simulink model "final"  (R2015a)
settings: Solver=FixedStepDiscrete  SolverMode=SingleTasking  StartTime=0.0  StopTime=3  RelTol=1e-3
PreLoadFcn:
  | Ts_Power=1e-6
  | Ts_Control=100e-6
values from neighbouring files (symbols this model uses):
  Iph_array = Iph*Npar    (= 29.801)    [sunpower305.m]
  Isat_array = Isat*Npar    (= 5.8765e-08)    [sunpower305.m]
  Rp_array = Rp*Nser/Npar    (= 198.702)    [sunpower305.m]
  Rs_array = Rs*Nser/Npar    (= 0.0075996)    [sunpower305.m]
  Ts = Ts_Power    (= 1e-06)    [sunpower305.m]
  VT_array = VT*Nser    (= 3.20466023218)    [sunpower305.m]
undefined symbols (not defined in the file or in its folder): D1, Delta, level, sigbuilder_block
libraries: powerlib x29, powerlib_extras x6, simulink x4
(part 1 of 2)
settings Model: SimulationMode=accelerator  Creator=Rupesh  LastModifiedBy=Limon
settings DataIOCC: SignalLoggingSaveFormat=ModelDataLogs
settings OptimizationCC: ExpressionDepthLimit=2147483647
settings DebuggingCC: UnderspecifiedInitializationDetection=Classic  MergeDetectMultiDrivingBlocksExec=none  SolverPrmCheckMsg=warning  FcnCallInpInsideContextMsg=EnableAllAsWarning  StateNameClashWarn=warning
settings GRTTargetCC: CombineOutputUpdateFcns=off  GRTInterface=on

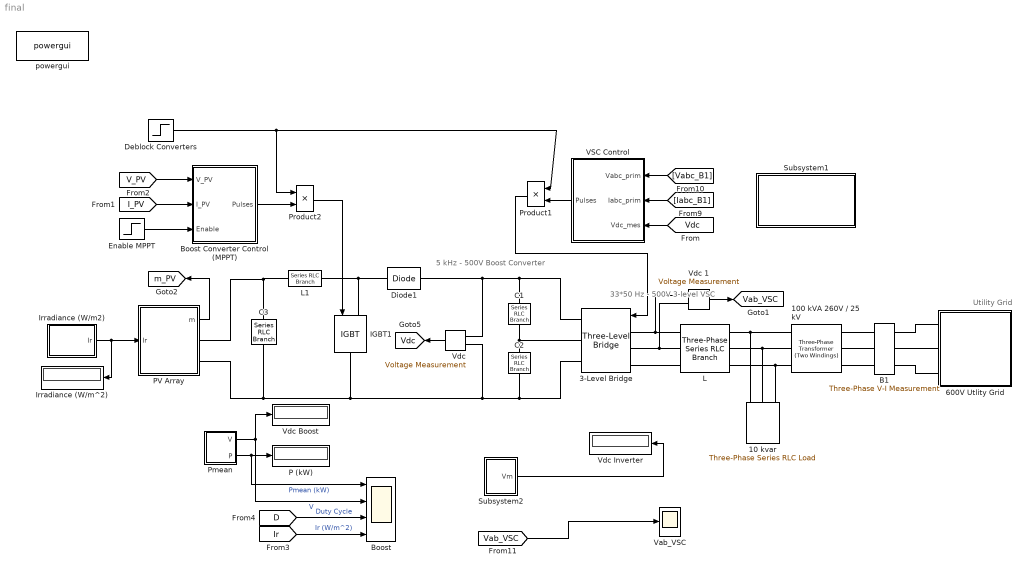
== system final ==
  note: 5 kHz - 500V
      | Boost Converter
  note: 33*50 Hz - 500V
      | 3-level VSC
  note: Utility Grid
  10 kvar : powerlib/Elements/Three-Phase Series RLC Load  LConnTagsString=A|B|C  Configuration=Y (grounded)  NominalVoltage=260  NominalFrequency=60  ActivePower=10e3/100  InductivePower=0  CapacitivePower=10e3  Measurements=None  LoadType=constant Z
  100 kVA 260V / 25 kV : powerlib/Elements/Three-Phase Transformer (Two Windings)  Winding1Connection=Yg  Winding2Connection=Delta (D1)  CoreType=Three single-phase transformers  SetSaturation=off  Hysteresis=off  DataFile='hysteresis'  SetInitialFlux=off  Measurements=None  UNITS=pu  NominalPower=[100e3 , 60 ]  Winding1=[ 25e3 , 0.001 , 0.03 ]  Winding2=[ 260 , 0.001 , 0.03 ]  Rm=500  Lm=500  L0=0.5  Saturation=[ 0,0 ; 0.0024,1.2 ; 1.0,1.52 ]  InitialFluxes=[ 0.8 , -0.8 , 0.7 ]  MoreParameters=off  BreakLoop=off  DataType=off  TransfoNumber=0
  3-Level Bridge : powerlib/Power Electronics/Three-Level Bridge  Arms=3  SnubberResistance=1e6  SbubberCapacitance=inf  Device=IGBT / Diodes  Ron=0.2e-3  ForwardVoltages="[  0  0 ]"  Measurements=None
  600V Utlity Grid : Subsystem
  B1 : powerlib/Measurements/Three-Phase V-I Measurement  VoltageMeasurement=phase-to-ground  SetLabelV=on  LabelV=Vabc_B1  Vpu=off  VpuLL=off  CurrentMeasurement=yes  SetLabelI=on  LabelI=Iabc_B1  Ipu=off  Pbase=100e6  Vbase=500e3  OutputType=Magnitude  PhasorSimulation=off  PSBequivalent=0
  Boost : Scope  NumInputPorts=4
      settings: TimeRange=3  YMin=0~0~0~200  YMax=17.5~800~0.5~1000  SaveName=ScopeData_Boost  Decimation=100  SampleInput=on  SampleTime=Ts_Control
  Boost Converter Control (MPPT) : Subsystem
  C1 : powerlib/Elements/Series RLC Branch  LConnTagsString=__new0  RConnTagsString=__new0  BranchType=C  Resistance=1.0  Inductance=1.0  SetiL0=off  InitialCurrent=0  Capacitance=1200e-06  Setx0=off  InitialVoltage=0  Measurements=None
  C2 : powerlib/Elements/Series RLC Branch  LConnTagsString=__new0  RConnTagsString=__new0  BranchType=C  Resistance=1.0  Inductance=1.0  SetiL0=off  InitialCurrent=0  Capacitance=1200e-06  Setx0=off  InitialVoltage=0  Measurements=None
  C3 : powerlib/Elements/Series RLC Branch  LConnTagsString=__new0  RConnTagsString=__new0  BranchType=C  Resistance=1.0  Inductance=1.0  SetiL0=off  InitialCurrent=0  Capacitance=100e-6  Setx0=off  InitialVoltage=0  Measurements=Branch voltage
  Deblock Converters : Step  Time=0.05  SampleTime=0
  Diode1 : powerlib/Power Electronics/Diode  Ron=1e-4  Lon=0  Vf=0  IC=0  UseSnubber=off  Rs=inf  Cs=inf  Measurements=off
  Enable MPPT : Step  Time=0.4  SampleTime=0
  IGBT1 : powerlib/Power Electronics/IGBT  Ron=0.001  Lon=0  Vf=0  Tf=0  Tt=0  IC=0  Rs=1e5  Cs=inf  Measurements=off
  "Irradiance (W/m2) " : Subsystem  Tag=STV Subsys  LoadFcn=sigbuilder_block('load');  StartFcn=sigbuilder_block('start');  StopFcn=sigbuilder_block('stop');  ClipboardFcn=sigbuilder_block('clipboard');  mask(Sigbuilder block){}
      mask help: Sigbuilder GUI
      mask init:
      | if ~strcmp(get_param(bdroot(gcbh),'SimulationStatus'),'stopped') tuvar = sigbuilder_block('maskInit'); end
      settings: CopyFcn=sigbuilder_block('copy');  DeleteFcn=sigbuilder_block('delete');  ModelCloseFcn=sigbuilder_block('modelClose');  PreSaveFcn=sigbuilder_block('preSave');  PauseFcn=sigbuilder_block('pause')  ContinueFcn=sigbuilder_block('continue')  NameChangeFcn=sigbuilder_block('namechange');  OpenFcn=sigbuilder_block('open',[9 136.5 954 513.75 ]);  CloseFcn=sigbuilder_block('close');
      mask Display: plot(0,0,100,100,[10,10,40,40,10],[80,20,20,80,80],[40,10],[50,50], [40,27,10],[65,72,56],[40,25,25,10],[28,28,43,43]);
  Irradiance (W/m^2) : Display
      settings: Format=bank  Decimation=1000
  L : powerlib/Elements/Three-Phase Series RLC Branch  LConnTagsString=A|B|C  RConnTagsString=A|B|C  BranchType=RL  Resistance=2e-3  Inductance=250e-6  Capacitance=inf  Measurements=None
  L1 : powerlib/Elements/Series RLC Branch  LConnTagsString=__new0  RConnTagsString=__new0  BranchType=RL  Resistance=0.005  Inductance=5e-3  SetiL0=off  InitialCurrent=0  Capacitance=1e-6  Setx0=off  InitialVoltage=0  Measurements=None
  "P (kW) " : Display
      settings: Format=bank  Decimation=2000
  PV Array : Subsystem
  Pmean : Subsystem
  Product1 : Product  RndMeth=Zero
  Product2 : Product  RndMeth=Zero
  Subsystem1 : Subsystem
      mask Display: disp('Measurements')
  Subsystem2 : Subsystem
  VSC Control : Subsystem  mask(VSC Main Controller){nom=[ 100e3  50 ], Vnom=[ 125e3 260 ], Vnom_dc=500, RLxfo=[0.002  0.06 ], RLchoke=[2e-3  250e-6  ], K_VDCreg=[7  800], K_Ireg=[0.3 20], Ts=Ts_Control}
      mask prompts: nom "Nominal power and frequency [ Pnom(VA)  Fnom(Hz) ]:"; Vnom "Nominal primary and secondary voltages (Vrms LL) [ Vnom_prim   Vnom_sec ]:"; Vnom_dc "Nominal DC bus voltage (V):"; RLxfo "Total transformer leakage impedance (pu/Pnom) [ Rxfo  Lxf ]"; RLchoke "Choke impedance [ R(ohm) L(H) ]"; K_VDCreg "VDC regultator gains [ Kp  Ki ]:"; K_Ireg "Current regulator gains [ Kp  Ki ]:"; Ts "Sample time"
      mask init:
      | Pnom=nom(1);
      | Fnom=nom(2);
      | Vnom_prim=Vnom(1);
      | Vnom_sec=Vnom(2);
      | Zbase=Vnom_sec^2/Pnom;
      | Rtot_pu=RLxfo(1) + RLchoke(1)/Zbase;
      | Ltot_pu=RLxfo(2) + RLchoke(2)/(Zbase/(2*pi*Fnom));
      | Kp_VDCreg=K_VDCreg(1);
      | Ki_VDCreg=K_VDCreg(2);
      | Kp_Ireg=K_Ireg(1);
      | Ki_Ireg=K_Ireg(2);
      | Vdc_ref=Vnom_dc;
  Vab_VSC : Scope
      settings: TimeRange=0.051  YMin=-1250  YMax=1250  SaveName=ScopeData7  Decimation=10
  "Vdc " : powerlib/Measurements/Voltage Measurement  Tag=PoWeRsYsTeMmEaSuReMeNt  PhasorSimulation=off  OutputType=Magnitude  PSBequivalent=0
  Vdc 1 : powerlib/Measurements/Voltage Measurement  Tag=PoWeRsYsTeMmEaSuReMeNt  PhasorSimulation=off  OutputType=Magnitude  PSBequivalent=0
  Vdc Boost : Display
      settings: Format=bank  Decimation=2000
  Vdc Inverter : Display
      settings: Format=bank  Decimation=2000
  powergui : powerlib/powergui  Priority=1  SimulationMode=Discrete  SolverType=Tustin  SampleTime=Ts_Power  frequency=60  SPID=off  DisableSnubberDevices=off  DisableRonSwitches=off  DisableVfSwitches=off  SwTol=0  DisplayEquations=off  Interpol=off  methode=off  Ts=0  FunctionMessages=off  echomessages=off  HookPort=off  EnableUseOfTLC=off  x0status=blocks  frequencyindice=0  Pbase=100e6  ErrMax=1e-4  Iterations=50  UnitsV=kV  UnitsW=MW  buscounter=0  RestoreLinks=warning  ResistiveCurrentMeasurement=off  Frange=[0:2:500]  Ylog=off  Xlog=on  ShowGrid=off  save=off  variable=ZData  structure=0  ZoomFFT=on  StartTime=0.0  cycles=1  DisplayStyle=1  fundamental=60  FreqAxis=off  MaxFrequency=1000  frequencyindicesteady=1  RmsSteady=1  display=off
  tag scope: Vab_VSC=global, Vdc=global, m_PV=global
  wires:
  "Vdc "/1 -> [Vdc]
  "Irradiance (W/m2) "/1(Ir) -> PV Array/1(Ir), Irradiance (W/m^2)/1
  Product2/1 -> IGBT1/1
  Deblock Converters/1 -> Product2/1, Product1/1
  [Iabc_B1] -> VSC Control/2(Iabc_prim)
  [Vdc] -> VSC Control/3(Vdc_mes)
  VSC Control/1(Pulses) -> Product1/2
  Product1/1 -> 3-Level Bridge/1
  Pmean/2(P) -> "P (kW) "/1, Boost/1  "Pmean (kW)"
  Vdc 1/1 -> [Vab_VSC]
  [Vab_VSC] -> Vab_VSC/1
  Pmean/1(V) -> Vdc Boost/1, Boost/2  "V"
  [D] -> Boost/3  "Duty Cycle"
  [Ir] -> Boost/4  "Ir (W/m^2)"
  Subsystem2/1(Vm) -> Vdc Inverter/1
  Boost Converter Control (MPPT)/1(Pulses) -> Product2/2
  [V_PV] -> Boost Converter Control (MPPT)/1(V_PV)
  [I_PV] -> Boost Converter Control (MPPT)/2(I_PV)
  Enable MPPT/1 -> Boost Converter Control (MPPT)/3(Enable)
  PV Array/1(m) -> [m_PV]
  [Vabc_B1] -> VSC Control/1(Vabc_prim)
  connections:
  Diode1/RConn1 -- 3-Level Bridge/RConn1 -- C1/LConn1 -- "Vdc "/LConn1
  L1/RConn1 -- Diode1/LConn1 -- IGBT1/LConn1
  3-Level Bridge/RConn3 -- C2/RConn1 -- "Vdc "/LConn2 -- C3/RConn1 -- PV Array/RConn2 -- IGBT1/RConn1
  3-Level Bridge/LConn1 -- L/LConn1 -- Vdc 1/LConn1
  3-Level Bridge/LConn2 -- L/LConn2 -- Vdc 1/LConn2
  3-Level Bridge/LConn3 -- L/LConn3
  L/RConn1 -- 100 kVA 260V / 25 kV/RConn1 -- 10 kvar/LConn1
  L/RConn2 -- 100 kVA 260V / 25 kV/RConn2 -- 10 kvar/LConn2
  L/RConn3 -- 100 kVA 260V / 25 kV/RConn3 -- 10 kvar/LConn3
  B1/LConn1 -- 100 kVA 260V / 25 kV/LConn1
  B1/LConn2 -- 100 kVA 260V / 25 kV/LConn2
  B1/LConn3 -- 100 kVA 260V / 25 kV/LConn3
  C2/LConn1 -- C1/RConn1 -- 3-Level Bridge/RConn2
  C3/LConn1 -- PV Array/RConn1 -- L1/LConn1
  B1/RConn2 -- 600V Utlity Grid/LConn2
  B1/RConn1 -- 600V Utlity Grid/LConn1
  B1/RConn3 -- 600V Utlity Grid/LConn3

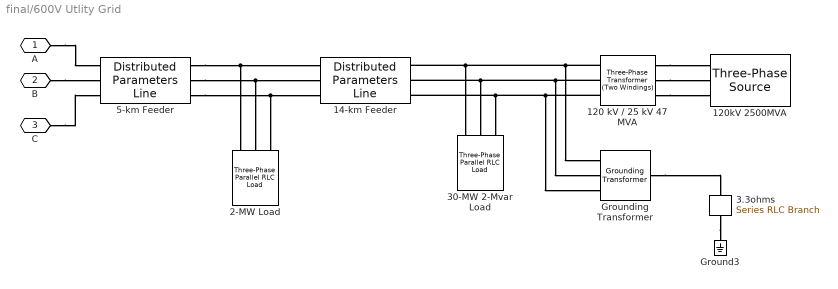
== system final/600V Utlity Grid ==
  120 kV / 25 kV 47 MVA : powerlib/Elements/Three-Phase Transformer (Two Windings)  Winding1Connection=Yg  Winding2Connection=Delta (D1)  CoreType=Three single-phase transformers  SetSaturation=off  Hysteresis=off  DataFile='basic_model'  SetInitialFlux=off  Measurements=None  UNITS=pu  NominalPower=[47e6 60 ]  Winding1="[ 120e3  0.08/30   0.08 ]"  Winding2="[ 25e3  0.08/30  0.08]"  Rm=500  Lm=500  L0=0.5  Saturation="[ 0,0  ;  0.005,1.2  ;  1.0,1.4 ]"  InitialFluxes=[ 0.8 , -0.8 , 0.7 ]  MoreParameters=off  BreakLoop=off  DataType=off  TransfoNumber=0
  120kV 2500MVA : powerlib/Electrical Sources/Three-Phase Source  Voltage=120e3  PhaseAngle=0  Frequency=60  InternalConnection=Yg  SpecifyImpedance=on  Resistance=0.8929  Inductance=16.58e-3  ShortCircuitLevel=2500e6  BaseVoltage=120e3  XRratio=7  BusType=swing  Pref=0  Qref=0  Qmin=-inf  Qmax=inf
  14-km Feeder : powerlib/Elements/Distributed Parameters Line  Phases=3  Frequency=60  Resistance=[0.1153 0.413]  Inductance=[1.05e-3 3.32e-3]  Capacitance=[11.33e-009 5.01e-009]  Length=14  x1=[-5.8e-05 -2.66241288531843e-10 0 0;-5.7e-05 -2.65838779606365e-10 0 0;-5.6e-05 -2.65436232899268e-10 0 0;-5.5e-05 -2.65033648467762e-10 0 0;-5.4e-05 -2.64631026369064e-10 0 0;-5.3e-05 -2.64228366660395e-10 0 0;-5.2e-05 -2.63825669398983e-10 0 0;-5.1e-05 -2.6342293464206e-10 0 0;-5e-05 -2.63020162446862e-10 0 0;-4.9e-05 -2.62617352870634e-10 -3790.5008820905 -24060.9143986523;-4.8e-05 -2.62214505970623e-10 -3781.42986191839 -24062.3416739891;-4.7e-05 -2.61811621804083e-10 -3772.35830432076 -24063.7655295306;-4.6e-05 -2.61408700428273e-10 -3763.28621058689 -24065.1859650743;-4.5e-05 -2.61005741900457e-10 -3754.21358200612 -24066.6029804184;-4.4e-05 -2.60602746277904e-10 -3745.14041986787 -24068.0165753614;-4.3e-05 -2.60199713617888e-10 -3736.06672546165 -24069.4267497026;-4.2e-05 -2.59796643977691e-10 -3726.99250007703 -24070.8335032414;-4.1e-05 -2.59393537414596e-10 -3717.91774500365 -24072.236835778;-4e-05 -2.58990393985895e-10 -3708.84246153125 -24073.6367471129;-3.9e-05 -2.58587213748883e-10 -3699.76665094961 -24075.0332370471;-3.8e-05 -2.58183996760861e-10 -3690.69031454863 -24076.4263053822;-3.7e-05 -2.57780743079135e-10 -3681.61345361825 -24077.8159519201;-3.6e-05 -2.57377452761016e-10 -3672.53606944848 -24079.2021764634;-3.5e-05 -2.56974125863822e-10 -3663.45816332944 -24080.5849788151;-3.4e-05 -2.56570762444873e-10 -3654.37973655129 -24081.9643587786;-3.3e-05 -2.56167362561497e-10 -3645.30079040428 -24083.340316158;-3.2e-05 -2.55763926271026e-10 -3636.22132617873 -24084.7128507575;-3.1e-05 -2.55360453630797e-10 -3627.14134516504 -24086.0819623823;-3e-05 -2.54956944698152e-10 -3618.06084865367 -24087.4476508376;-2.9e-05 -2.5455339953044e-10 -3608.97983793517 -24088.8099159294;-2.8e-05 -2.54149818185012e-10 -3599.89831430014 -24090.1687574641;-2.7e-05 -2.53746200719228e-10 -3590.81627903928 -24091.5241752486;-2.6e-05 -2.53342547190449e-10 -3581.73373344335 -24092.8761690902;-2.5e-05 -2.52938857656045e-10 -3572.65067880317 -24094.2247387968;-2.4e-05 -2.52535132173387e-10 -3563.56711640966 -24095.5698841767;-2.3e-05 -2.52131370799856e-10 -3554.48304755378 -24096.9116050388;-2.2e-05 -2.51727573592834e-10 -3545.3984735266 -24098.2499011923;-2.1e-05 -2.51323740609709e-10 -3536.31339561922 -24099.5847724471;-2e-05 -2.50919871907877e-10 -3527.22781512284 -24100.9162186135;-1.9e-05 -2.50515967544734e-10 -3518.14173332873 -24102.2442395021;-1.8e-05 -2.50112027577686e-10 -3509.05515152821 -24103.5688349243;-1.7e-05 -2.4970805206414e-10 -3499.9680710127 -24104.8900046919;-1.6e-05 -2.49304041061511e-10 -3490.88049307368 -24106.2077486169;-1.5e-05 -2.48899994627219e-10 -3481.79241900268 -24107.5220665123;-1.4e-05 -2.48495912818686e-10 -3472.70385009133 -24108.8329581911;-1.3e-05 -2.48091795693342e-10 -3463.61478763132 -24110.1404234671;-1.2e-05 -2.47687643308621e-10 -3454.52523291439 -24111.4444621545;-1.1e-05 -2.47283455721962e-10 -3445.4351872324 -24112.7450740678;-1e-05 -2.46879232990809e-10 -3436.34465187722 -24114.0422590224;-9e-06 -2.46474975172611e-10 -3427.25362814083 -24115.3360168337;-8e-06 -2.46070682324823e-10 -3418.16211731527 -24116.626347318;-7e-06 -2.45666354504902e-10 -3409.07012069264 -24117.9132502918;-6e-06 -2.45261991770314e-10 -3399.97763956512 -24119.1967255723;-5e-06 -2.44857594178528e-10 -3390.88467522495 -24120.4767729771;-4e-06 -2.44453161787016e-10 -3381.79122896444 -24121.7533923241;-3e-06 -2.44048694653258e-10 -3372.69730207598 -24123.0265834321;-2e-06 -2.43644192834738e-10 -3363.60289585202 -24124.29634612;-1e-06 -2.43239656388945e-10 -3354.50801158508 -24125.5626802074]  x2=[-5.8e-05 -2.19441538908334e-10 0 0;-5.7e-05 -2.19014640734556e-10 0 0;-5.6e-05 -2.18587711433914e-10 0 0;-5.5e-05 -2.18160751067083e-10 0 0;-5.4e-05 -2.17733759694744e-10 0 0;-5.3e-05 -2.17306737377582e-10 0 0;-5.2e-05 -2.16879684176287e-10 0 0;-5.1e-05 -2.16452600151551e-10 0 0;-5e-05 -2.16025485364074e-10 0 0;-4.9e-05 -2.15598339874557e-10 -3379.33798532399 -24243.9018981772;-4.8e-05 -2.15171163743709e-10 -3370.19800970911 -24245.1741557541;-4.7e-05 -2.14743957032239e-10 -3361.05755511394 -24246.4429675511;-4.6e-05 -2.14316719800863e-10 -3351.91662283753 -24247.7083333877;-4.5e-05 -2.13889452110303e-10 -3342.77521417902 -24248.9702530843;-4.4e-05 -2.1346215402128e-10 -3333.6333304376 -24250.2287264613;-4.3e-05 -2.13034825594526e-10 -3324.49097291254 -24251.4837533401;-4.2e-05 -2.12607466890771e-10 -3315.34814290317 -24252.7353335421;-4.1e-05 -2.12180077970754e-10 -3306.20484170889 -24253.9834668896;-4e-05 -2.11752658895216e-10 -3297.06107062916 -24255.2281532052;-3.9e-05 -2.11325209724903e-10 -3287.91683096353 -24256.4693923119;-3.8e-05 -2.10897730520564e-10 -3278.7721240116 -24257.7071840333;-3.7e-05 -2.10470221342955e-10 -3269.62695107302 -24258.9415281935;-3.6e-05 -2.10042682252833e-10 -3260.48131344753 -24260.1724246172;-3.5e-05 -2.09615113310962e-10 -3251.33521243493 -24261.3998731293;-3.4e-05 -2.09187514578108e-10 -3242.18864933509 -24262.6238735554;-3.3e-05 -2.08759886115043e-10 -3233.04162544794 -24263.8444257215;-3.2e-05 -2.08332227982543e-10 -3223.89414207347 -24265.0615294542;-3.1e-05 -2.07904540241387e-10 -3214.74620051174 -24266.2751845806;-3e-05 -2.0747682295236e-10 -3205.59780206289 -24267.485390928;-2.9e-05 -2.07049076176248e-10 -3196.44894802709 -24268.6921483246;-2.8e-05 -2.06621299973846e-10 -3187.29963970462 -24269.8954565988;-2.7e-05 -2.06193494405948e-10 -3178.14987839578 -24271.0953155796;-2.6e-05 -2.05765659533357e-10 -3168.99966540097 -24272.2917250964;-2.5e-05 -2.05337795416877e-10 -3159.84900202063 -24273.4846849793;-2.4e-05 -2.04909902117316e-10 -3150.69788955528 -24274.6741950587;-2.3e-05 -2.04481979695488e-10 -3141.54632930549 -24275.8602551655;-2.2e-05 -2.04054028212211e-10 -3132.3943225719 -24277.0428651311;-2.1e-05 -2.03626047728306e-10 -3123.24187065523 -24278.2220247876;-2e-05 -2.03198038304598e-10 -3114.08897485623 -24279.3977339673;-1.9e-05 -2.02770000001917e-10 -3104.93563647574 -24280.569992503;-1.8e-05 -2.02341932881097e-10 -3095.78185681465 -24281.7388002283;-1.7e-05 -2.01913837002976e-10 -3086.62763717392 -24282.904156977;-1.6e-05 -2.01485712428396e-10 -3077.47297885456 -24284.0660625834;-1.5e-05 -2.01057559218202e-10 -3068.31788315766 -24285.2245168825;-1.4e-05 -2.00629377433246e-10 -3059.16235138436 -24286.3795197096;-1.3e-05 -2.0020116713438e-10 -3050.00638483587 -24287.5310709005;-1.2e-05 -1.99772928382464e-10 -3040.84998481345 -24288.6791702916;-1.1e-05 -1.99344661238359e-10 -3031.69315261842 -24289.8238177197;-1e-05 -1.98916365762932e-10 -3022.53588955219 -24290.9650130221;-9e-06 -1.98488042017054e-10 -3013.37819691621 -24292.1027560367;-8e-06 -1.98059690061598e-10 -3004.22007601197 -24293.2370466017;-7e-06 -1.97631309957443e-10 -2995.06152814107 -24294.367884556;-6e-06 -1.97202901765471e-10 -2985.90255460513 -24295.4952697388;-5e-06 -1.9677446554657e-10 -2976.74315670584 -24296.6192019898;-4e-06 -1.96346001361628e-10 -2967.58333574496 -24297.7396811495;-3e-06 -1.9591750927154e-10 -2958.42309302431 -24298.8567070584;-2e-06 -1.95488989337205e-10 -2949.26242984576 -24299.9702795579;-1e-06 -1.95060441619526e-10 -2940.10134751125 -24301.0803984897]  x3=[-5.8e-05 -2.83245009916326e-12 0 0;-5.7e-05 -2.83025796249545e-12 0 0;-5.6e-05 -2.82806542358487e-12 0 0;-5.5e-05 -2.82587248274312e-12 0 0;-5.4e-05 -2.82367914028187e-12 0 0;-5.3e-05 -2.82148539651284e-12 0 0;-5.2e-05 -2.81929125174781e-12 0 0;-5.1e-05 -2.81709670629862e-12 0 0;-5e-05 -2.81490176047716e-12 0 0;-4.9e-05 -2.81270641459538e-12 -23.610210034582 -155.666879550889;-4.8e-05 -2.8105106689653e-12 -23.5515233271788 -155.675769328298;-4.7e-05 -2.80831452389897e-12 -23.492833272579 -155.684636980708;-4.6e-05 -2.80611797970851e-12 -23.4341398791236 -155.69348250686;-4.5e-05 -2.80392103670611e-12 -23.3754431551543 -155.702305905495;-4.4e-05 -2.801723695204e-12 -23.3167431090132 -155.71110717536;-4.3e-05 -2.79952595551447e-12 -23.258039749043 -155.719886315204;-4.2e-05 -2.79732781794986e-12 -23.1993330835866 -155.728643323779;-4.1e-05 -2.79512928282259e-12 -23.1406231209875 -155.737378199842;-4e-05 -2.79293035044511e-12 -23.0819098695899 -155.746090942149;-3.9e-05 -2.79073102112994e-12 -23.0231933377381 -155.754781549464;-3.8e-05 -2.78853129518965e-12 -22.9644735337771 -155.763450020551;-3.7e-05 -2.78633117293688e-12 -22.9057504660522 -155.772096354177;-3.6e-05 -2.7841306546843e-12 -22.8470241429094 -155.780720549115;-3.5e-05 -2.78192974074468e-12 -22.7882945726948 -155.789322604138;-3.4e-05 -2.77972843143079e-12 -22.7295617637555 -155.797902518024;-3.3e-05 -2.7775267270555e-12 -22.6708257244385 -155.806460289554;-3.2e-05 -2.77532462793172e-12 -22.6120864630915 -155.81499591751;-3.1e-05 -2.77312213437241e-12 -22.5533439880628 -155.823509400681;-3e-05 -2.77091924669061e-12 -22.4945983077009 -155.832000737857;-2.9e-05 -2.76871596519938e-12 -22.4358494303549 -155.840469927829;-2.8e-05 -2.76651229021187e-12 -22.3770973643744 -155.848916969395;-2.7e-05 -2.76430822204126e-12 -22.3183421181093 -155.857341861355;-2.6e-05 -2.76210376100081e-12 -22.25958369991 -155.86574460251;-2.5e-05 -2.75989890740381e-12 -22.2008221181275 -155.874125191667;-2.4e-05 -2.75769366156362e-12 -22.142057381113 -155.882483627634;-2.3e-05 -2.75548802379367e-12 -22.0832894972184 -155.890819909224;-2.2e-05 -2.75328199440742e-12 -22.0245184747958 -155.899134035252;-2.1e-05 -2.75107557371839e-12 -21.965744322198 -155.907426004536;-2e-05 -2.74886876204017e-12 -21.9069670477781 -155.915695815898;-1.9e-05 -2.74666155968639e-12 -21.8481866598895 -155.923943468163;-1.8e-05 -2.74445396697075e-12 -21.7894031668864 -155.932168960157;-1.7e-05 -2.742245984207e-12 -21.7306165771231 -155.940372290713;-1.6e-05 -2.74003761170893e-12 -21.6718268989546 -155.948553458664;-1.5e-05 -2.73782884979042e-12 -21.6130341407362 -155.956712462848;-1.4e-05 -2.73561969876536e-12 -21.5542383108236 -155.964849302105;-1.3e-05 -2.73341015894774e-12 -21.4954394175731 -155.972963975279;-1.2e-05 -2.73120023065157e-12 -21.4366374693413 -155.981056481216;-1.1e-05 -2.72898991419094e-12 -21.3778324744851 -155.989126818766;-1e-05 -2.72677920987998e-12 -21.3190244413623 -155.997174986782;-9e-06 -2.72456811803289e-12 -21.2602133783306 -156.005200984121;-8e-06 -2.7223566389639e-12 -21.2013992937484 -156.013204809642;-7e-06 -2.72014477298732e-12 -21.1425821959746 -156.021186462207;-6e-06 -2.71793252041751e-12 -21.0837620933683 -156.029145940681;-5e-06 -2.71571988156887e-12 -21.0249389942892 -156.037083243935;-4e-06 -2.71350685675587e-12 -20.9661129070974 -156.044998370839;-3e-06 -2.71129344629303e-12 -20.9072838401534 -156.052891320268;-2e-06 -2.70907965049492e-12 -20.8484518018181 -156.060762091102;-1e-06 -2.70686546967618e-12 -20.7896168004528 -156.06861068222]  x4=[-5.8e-05 1.99167322087456e-12 0 0;-5.7e-05 1.99117155346646e-12 0 0;-5.6e-05 1.99066960306846e-12 0 0;-5.5e-05 1.99016736975192e-12 0 0;-5.4e-05 1.98966485358822e-12 0 0;-5.3e-05 1.98916205464876e-12 0 0;-5.2e-05 1.98865897300502e-12 0 0;-5.1e-05 1.98815560872849e-12 0 0;-5e-05 1.9876519618907e-12 0 0;-4.9e-05 1.98714803256324e-12 -1.28892375628843 -2.16547060902882;-4.8e-05 1.98664382081773e-12 -1.28810730152854 -2.16595636794494;-4.7e-05 1.98613932672583e-12 -1.28729066369987 -2.16644181903035;-4.6e-05 1.98563455035924e-12 -1.28647384291849 -2.16692696221606;-4.5e-05 1.98512949178969e-12 -1.28565683930048 -2.16741179743312;-4.4e-05 1.98462415108897e-12 -1.28483965296197 -2.16789632461263;-4.3e-05 1.9841185283289e-12 -1.28402228401909 -2.16838054368573;-4.2e-05 1.98361262358133e-12 -1.283204732588 -2.16886445458359;-4.1e-05 1.98310643691818e-12 -1.28238699878491 -2.16934805723744;-4e-05 1.98259996841137e-12 -1.28156908272602 -2.16983135157855;-3.9e-05 1.98209321813289e-12 -1.28075098452758 -2.17031433753824;-3.8e-05 1.98158618615476e-12 -1.27993270430587 -2.17079701504786;-3.7e-05 1.98107887254904e-12 -1.27911424217717 -2.17127938403881;-3.6e-05 1.98057127738783e-12 -1.27829559825782 -2.17176144444254;-3.5e-05 1.98006340074328e-12 -1.27747677266415 -2.17224319619053;-3.4e-05 1.97955524268755e-12 -1.27665776551254 -2.17272463921432;-3.3e-05 1.97904680329288e-12 -1.2758385769194 -2.17320577344548;-3.2e-05 1.97853808263152e-12 -1.27501920700113 -2.17368659881563;-3.1e-05 1.97802908077578e-12 -1.27419965587421 -2.17416711525645;-3e-05 1.97751979779799e-12 -1.27337992365509 -2.17464732269963;-2.9e-05 1.97701023377053e-12 -1.27256001046029 -2.17512722107692;-2.8e-05 1.97650038876583e-12 -1.27173991640633 -2.17560681032013;-2.7e-05 1.97599026285635e-12 -1.27091964160977 -2.17608609036109;-2.6e-05 1.97547985611458e-12 -1.27009918618718 -2.17656506113169;-2.5e-05 1.97496916861306e-12 -1.26927855025518 -2.17704372256385;-2.4e-05 1.97445820042439e-12 -1.26845773393038 -2.17752207458954;-2.3e-05 1.97394695162116e-12 -1.26763673732945 -2.17800011714079;-2.2e-05 1.97343542227606e-12 -1.26681556056907 -2.17847785014965;-2.1e-05 1.97292361246177e-12 -1.26599420376595 -2.17895527354822;-2e-05 1.97241152225103e-12 -1.26517266703682 -2.17943238726865;-1.9e-05 1.97189915171663e-12 -1.26435095049843 -2.17990919124313;-1.8e-05 1.97138650093138e-12 -1.26352905426758 -2.18038568540391;-1.7e-05 1.97087356996815e-12 -1.26270697846107 -2.18086186968325;-1.6e-05 1.97036035889983e-12 -1.26188472319574 -2.18133774401348;-1.5e-05 1.96984686779936e-12 -1.26106228858845 -2.18181330832697;-1.4e-05 1.96933309673972e-12 -1.26023967475608 -2.18228856255613;-1.3e-05 1.96881904579392e-12 -1.25941688181555 -2.18276350663342;-1.2e-05 1.96830471503503e-12 -1.2585939098838 -2.18323814049134;-1.1e-05 1.96779010453615e-12 -1.25777075907778 -2.18371246406242;-1e-05 1.9672752143704e-12 -1.25694742951448 -2.18418647727926;-9e-06 1.96676004461098e-12 -1.25612392131092 -2.1846601800745;-8e-06 1.96624459533109e-12 -1.25530023458414 -2.1851335723808;-7e-06 1.96572886660399e-12 -1.2544763694512 -2.18560665413089;-6e-06 1.96521285850298e-12 -1.2536523260292 -2.18607942525753;-5e-06 1.96469657110139e-12 -1.25282810443524 -2.18655188569353;-4e-06 1.96418000447261e-12 -1.25200370478646 -2.18702403537174;-3e-06 1.96366315869005e-12 -1.25117912720004 -2.18749587422506;-2e-06 1.96314603382715e-12 -1.25035437179315 -2.18796740218644;-1e-06 1.96262862995743e-12 -1.24952943868303 -2.18843861918885]  x5=5.70973484498186e-05  V1=ones(3,3)  V2=ones(3,3)  I1=ones(3,3)  I2=ones(3,3)  nHarmo=1  Measurements=None
  2-MW Load : powerlib/Elements/Three-Phase Parallel RLC Load  LConnTagsString=A|B|C  Configuration=Y (grounded)  NominalVoltage=25e3  NominalFrequency=60  ActivePower=2e6  InductivePower=0  CapacitivePower=0  Measurements=None  LoadType=constant Z
  "3.3ohms " : powerlib/Elements/Series RLC Branch  LConnTagsString=__new0  RConnTagsString=__new0  BranchType=R  Resistance=3.3  Inductance=[]  SetiL0=off  InitialCurrent=0  Capacitance=[]  Setx0=off  InitialVoltage=0  Measurements=None
  30-MW 2-Mvar Load : powerlib/Elements/Three-Phase Parallel RLC Load  LConnTagsString=A|B|C  Configuration=Y (grounded)  NominalVoltage=25e3  NominalFrequency=60  ActivePower=30e6  InductivePower=2e6  CapacitivePower=0  Measurements=None  LoadType=constant Z
  5-km Feeder : powerlib/Elements/Distributed Parameters Line  Phases=3  Frequency=60  Resistance=[0.1153 0.413]  Inductance=[1.05e-3 3.32e-3]  Capacitance=[11.33e-009 5.01e-009]  Length=5  x1=[-2.1e-05 -2.5034227216243e-10 -3536.88834563299 -24100.782456778;-2e-05 -2.49941829422639e-10 -3527.80231357941 -24102.1141196103;-1.9e-05 -2.4954135116054e-10 -3518.71578014645 -24103.4423569946;-1.8e-05 -2.49140837433051e-10 -3509.6287466255 -24104.7671687422;-1.7e-05 -2.48740288297092e-10 -3500.54121430803 -24106.0885546649;-1.6e-05 -2.4833970380959e-10 -3491.45318448559 -24107.4065145747;-1.5e-05 -2.47939084027478e-10 -3482.36465844979 -24108.7210482845;-1.4e-05 -2.47538429007693e-10 -3473.27563749231 -24110.0321556073;-1.3e-05 -2.47137738807177e-10 -3464.1861229049 -24111.3398363568;-1.2e-05 -2.46737013482877e-10 -3455.09611597938 -24112.6440903473;-1.1e-05 -2.46336253091744e-10 -3446.00561800765 -24113.9449173932;-1e-05 -2.45935457690736e-10 -3436.91463028167 -24115.2423173098;-9e-06 -2.45534627336814e-10 -3427.82315409348 -24116.5362899127;-8e-06 -2.45133762086946e-10 -3418.73119073516 -24117.8268350179;-7e-06 -2.44732861998104e-10 -3409.6387414989 -24119.113952442;-6e-06 -2.44331927127264e-10 -3400.54580767694 -24120.3976420022;-5e-06 -2.43930957531408e-10 -3391.45239056158 -24121.6779035159;-4e-06 -2.43529953267523e-10 -3382.35849144519 -24122.9547368013;-3e-06 -2.43128914392601e-10 -3373.26411162024 -24124.2281416768;-2e-06 -2.42727840963638e-10 -3364.16925237922 -24125.4981179614;-1e-06 -2.42326733037635e-10 -3355.07391501473 -24126.7646654748]  x2=[-2.1e-05 -2.51338141059124e-10 -3536.31339561922 -24099.5847724471;-2e-05 -2.50933586634924e-10 -3527.22781512284 -24100.9162186135;-1.9e-05 -2.50528996547465e-10 -3518.14173332873 -24102.2442395021;-1.8e-05 -2.50124370854249e-10 -3509.05515152821 -24103.5688349243;-1.7e-05 -2.49719709612781e-10 -3499.9680710127 -24104.8900046919;-1.6e-05 -2.49315012880574e-10 -3490.88049307368 -24106.2077486169;-1.5e-05 -2.48910280715143e-10 -3481.79241900268 -24107.5220665123;-1.4e-05 -2.4850551317401e-10 -3472.70385009133 -24108.8329581911;-1.3e-05 -2.48100710314701e-10 -3463.61478763132 -24110.1404234671;-1.2e-05 -2.47695872194748e-10 -3454.52523291439 -24111.4444621545;-1.1e-05 -2.47290998871688e-10 -3445.4351872324 -24112.7450740678;-1e-05 -2.46886090403062e-10 -3436.34465187722 -24114.0422590224;-9e-06 -2.46481146846417e-10 -3427.25362814083 -24115.3360168337;-8e-06 -2.46076168259303e-10 -3418.16211731527 -24116.626347318;-7e-06 -2.45671154699279e-10 -3409.07012069264 -24117.9132502918;-6e-06 -2.45266106223904e-10 -3399.97763956512 -24119.1967255723;-5e-06 -2.44861022890745e-10 -3390.88467522495 -24120.4767729771;-4e-06 -2.44455904757375e-10 -3381.79122896444 -24121.7533923241;-3e-06 -2.44050751881369e-10 -3372.69730207598 -24123.0265834321;-2e-06 -2.43645564320308e-10 -3363.60289585202 -24124.29634612;-1e-06 -2.43240342131778e-10 -3354.50801158508 -24125.5626802074]  x3=[-2.1e-05 -2.36505659627167e-12 -11.2236902755013 -79.1234381044686;-2e-05 -2.36496717365722e-12 -11.1938606452144 -79.1276637133157;-1.9e-05 -2.36487741492819e-12 -11.1640294240303 -79.1318780763571;-1.8e-05 -2.36478732009734e-12 -11.1341966161886 -79.1360811929938;-1.7e-05 -2.36469688917747e-12 -11.1043622259293 -79.1402730626285;-1.6e-05 -2.36460612218143e-12 -11.0745262574924 -79.1444536846655;-1.5e-05 -2.36451501912213e-12 -11.0446887151184 -79.1486230585106;-1.4e-05 -2.36442358001252e-12 -11.0148496030478 -79.1527811835711;-1.3e-05 -2.36433180486558e-12 -10.9850089255215 -79.1569280592562;-1.2e-05 -2.36423969369436e-12 -10.9551666867803 -79.1610636849766;-1.1e-05 -2.36414724651196e-12 -10.9253228910657 -79.1651880601443;-1e-05 -2.36405446333151e-12 -10.895477542619 -79.1693011841733;-9e-06 -2.36396134416619e-12 -10.865630645682 -79.173403056479;-8e-06 -2.36386788902925e-12 -10.8357822044966 -79.1774936764784;-7e-06 -2.36377409793397e-12 -10.8059322233048 -79.1815730435901;-6e-06 -2.36367997089367e-12 -10.7760807063491 -79.1856411572345;-5e-06 -2.36358550792173e-12 -10.746227657872 -79.1896980168332;-4e-06 -2.36349070903158e-12 -10.7163730821163 -79.1937436218099;-3e-06 -2.36339557423669e-12 -10.686516983325 -79.1977779715894;-2e-06 -2.36330010355058e-12 -10.6566593657412 -79.2018010655984;-1e-06 -2.36320429698682e-12 -10.6268002336086 -79.2058129032651]  x4=[-2.1e-05 7.7440198490703e-13 -12.4922083172047 -78.9091123636771;-2e-05 7.7469853203757e-13 -12.4624593956743 -78.9138162077783;-1.9e-05 7.74994969066172e-13 -12.4327087029504 -78.9185088364664;-1.8e-05 7.75291295950704e-13 -12.4029562432614 -78.9231902490744;-1.7e-05 7.75587512649053e-13 -12.3732020208357 -78.9278604449369;-1.6e-05 7.7588361911912e-13 -12.3434460399021 -78.9325194233902;-1.5e-05 7.76179615318821e-13 -12.3136883046895 -78.9371671837722;-1.4e-05 7.76475501206088e-13 -12.2839288194271 -78.9418037254223;-1.3e-05 7.7677127673887e-13 -12.2541675883445 -78.9464290476816;-1.2e-05 7.77066941875131e-13 -12.2244046156715 -78.9510431498926;-1.1e-05 7.77362496572848e-13 -12.1946399056379 -78.9556460313997;-1e-05 7.77657940790019e-13 -12.164873462474 -78.9602376915486;-9e-06 7.77953274484653e-13 -12.1351052904103 -78.9648181296868;-8e-06 7.78248497614777e-13 -12.1053353936775 -78.9693873451633;-7e-06 7.78543610138434e-13 -12.0755637765065 -78.9739453373287;-6e-06 7.7883861201368e-13 -12.0457904431287 -78.9784921055352;-5e-06 7.79133503198591e-13 -12.0160153977754 -78.9830276491366;-4e-06 7.79428283651254e-13 -11.9862386446783 -78.9875519674884;-3e-06 7.79722953329776e-13 -11.9564601880694 -78.9920650599474;-2e-06 7.80017512192277e-13 -11.9266800321809 -78.9965669258724;-1e-06 7.80311960196894e-13 -11.8968981812451 -79.0010575646234]  x5=2.03919101606495e-05  V1=ones(3,3)  V2=ones(3,3)  I1=ones(3,3)  I2=ones(3,3)  nHarmo=1  Measurements=None
  Ground3 : powerlib/Elements/Ground  LConnTagsString=a
  "Grounding Transformer " : powerlib/Elements/Grounding Transformer   UNITS=pu  NominalPower="[100e6   60]"  NominalVoltage=25e3  ZeroSequenceImpedance_pu=[0.025 0.75]  MagnetizationBranch_pu=[500 500]  ZeroSequenceImpedance_SI=[0.052083 589.05]  MagnetizationBranch_SI=[1041.7 3.927e+005]  Measurements=None
  A : PMIOPort  Port=1  Side=Left
  B : PMIOPort  Port=2  Side=Left
  C : PMIOPort  Port=3  Side=Left
  connections:
  "3.3ohms "/RConn1 -- Ground3/LConn1
  120 kV / 25 kV 47 MVA/LConn1 -- 120kV 2500MVA/RConn1
  120 kV / 25 kV 47 MVA/LConn2 -- 120kV 2500MVA/RConn2
  120 kV / 25 kV 47 MVA/LConn3 -- 120kV 2500MVA/RConn3
  120 kV / 25 kV 47 MVA/RConn1 -- "Grounding Transformer "/LConn1 -- 14-km Feeder/RConn1 -- 30-MW 2-Mvar Load/LConn1
  120 kV / 25 kV 47 MVA/RConn2 -- "Grounding Transformer "/LConn2 -- 14-km Feeder/RConn2 -- 30-MW 2-Mvar Load/LConn2
  120 kV / 25 kV 47 MVA/RConn3 -- "Grounding Transformer "/LConn3 -- 14-km Feeder/RConn3 -- 30-MW 2-Mvar Load/LConn3
  5-km Feeder/RConn1 -- 14-km Feeder/LConn1 -- 2-MW Load/LConn1
  5-km Feeder/RConn2 -- 14-km Feeder/LConn2 -- 2-MW Load/LConn2
  5-km Feeder/RConn3 -- 14-km Feeder/LConn3 -- 2-MW Load/LConn3
  A/RConn1 -- 5-km Feeder/LConn1
  B/RConn1 -- 5-km Feeder/LConn2
  C/RConn1 -- 5-km Feeder/LConn3
  "Grounding Transformer "/RConn1 -- "3.3ohms "/LConn1

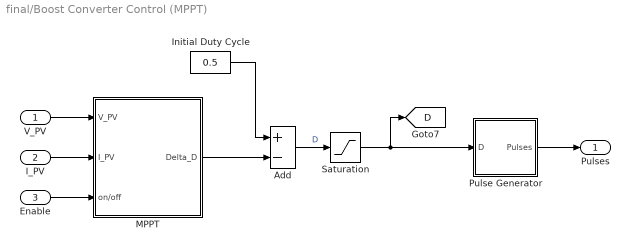
== system final/Boost Converter Control (MPPT) ==
  V_PV : Inport
  I_PV : Inport  Port=2
  Enable : Inport  Port=3
  Add : Sum  Inputs=+-
  Initial Duty Cycle : Constant  Value=0.5
  MPPT : Subsystem
  Pulse Generator : Subsystem  mask{Freq=5000}
      mask prompts: Freq "Frequency (Hz)"
  Saturation : Saturate  UpperLimit=1  LowerLimit=0
  Pulses : Outport
  tag scope: D=global
  wires:
  Initial Duty Cycle/1 -> Add/1
  MPPT/1(Delta_D) -> Add/2
  Add/1 -> Saturation/1  "D"
  Saturation/1 -> Pulse Generator/1(D), [D]
  Enable/1 -> MPPT/3(on/off)
  Pulse Generator/1(Pulses) -> Pulses/1
  I_PV/1 -> MPPT/2(I_PV)
  V_PV/1 -> MPPT/1(V_PV)

== system final/Irradiance (W//m2)  ==
  Demux : Demux  Tag=STV Demux  Outputs=1
  FromWs : FromWorkspace  Tag=STV FromWs  VariableName=tuvar  SampleTime=0
      SigBuilderData=|
      | common.afterFinalStr = 'Extrapolate'
      | common.sampleTime = '0'
      | dataSet(1).timeRange = [0 1]
      | dataSet(1).name = 'Constant Irradiance'
      | dataSet(2).timeRange = [0 1]
      | dataSet(2).name = 'Step Irradiance'
      | dataSet(3).timeRange = [0 3]
      | dataSet(3).name = 'Ramp-up/down Irradiance'
      | sbobj.Groups(1).Name = 'Constant Irradiance'
      | sbobj.Groups(1).Signals.Name = 'Ir'
      | sbobj.Groups(1).Signals.XData = [0 1]
      | sbobj.Groups(1).Signals.YData = [1000 1000]
      | sbobj.Groups(1).TimeRange = [0 1]
      | sbobj.Groups(2).Name = 'Step Irradiance'
      | sbobj.Groups(2).Signals.Name = 'Ir'
      | sbobj.Groups(2).Signals.XData = [0 0.501 0.51 0.69 0.7 1]
      | sbobj.Groups(2).Signals.YData = [1000 1000 250 250 1000 1000]
      | sbobj.Groups(2).TimeRange = [0 1]
      | sbobj.Groups(3).Name = 'Ramp-up/down Irradiance'
      | sbobj.Groups(3).Signals.Name = 'Ir'
      | sbobj.Groups(3).Signals.XData = [0 0.7 1.2 1.5 2 2.3 2.35 2.65 2.7 3]
      | sbobj.Groups(3).Signals.YData = [1000 1000 250 250 1000 1000 250 250 1000 1000]
      | sbobj.Groups(3).TimeRange = [0 3]
  Ir : Outport  Tag=STV Outport
  wires:
  Demux/1 -> Ir/1
  FromWs/1 -> Demux/1

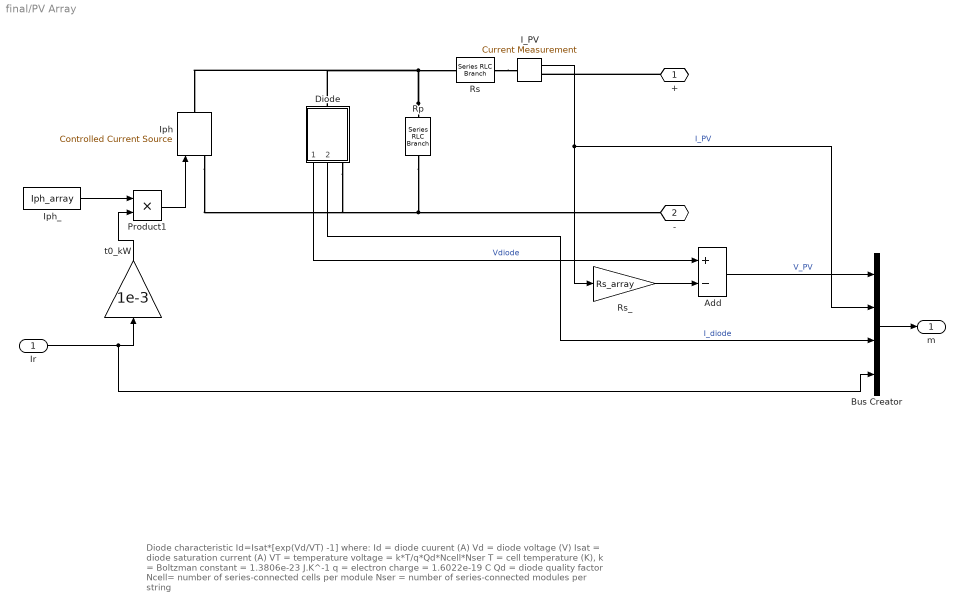
== system final/PV Array ==
  note: Diode characteristic
      | Id=Isat*[exp(Vd/VT) -1]
      |
      | where:
      | Id = diode cuurent (A)
      | Vd = diode voltage (V)
      | Isat = diode saturation current (A)
      | VT = temperature voltage = k*T/q*Qd*Ncell*Nser
      |
      | T = cell temperature (K),
      | k = Boltzman constant = 1.3806e-23 J.K^-1
      | q = electron charge = 1.6022e-19 C
      | Qd = diode quality factor
      | Ncell= number of series-connected cells per module
      | Nser = number of series-connected modules per string
  Ir : Inport
  Add : Sum  Inputs=+-
  Bus Creator : BusCreator
  Diode : Subsystem
      mask Display:
      | plot(-75,-50,100,150, [-15 -15 43 -15 -15 -75],[50 8 50 92 50 50], ...
      |     [43 43],[8 94],[100 43], [50 50])
  I_PV : powerlib/Measurements/Current Measurement  PhasorSimulation=off  OutputType=Complex  PSBequivalent=0
  Iph : powerlib/Electrical Sources/Controlled Current Source  Initialize=on  Source_Type=AC  Amplitude=0  Phase=0  Frequency=0  Measurements=None
  Iph_ : Constant  Value=Iph_array
  Product1 : Product  Inputs=**  RndMeth=Zero
  Rp : powerlib/Elements/Series RLC Branch  LConnTagsString=__new0  RConnTagsString=__new0  BranchType=R  Resistance=Rp_array  Inductance=1e-3  SetiL0=off  InitialCurrent=0  Capacitance=1e-6  Setx0=off  InitialVoltage=0  Measurements=Branch current
  Rs : powerlib/Elements/Series RLC Branch  LConnTagsString=__new0  RConnTagsString=__new0  BranchType=R  Resistance=Rs_array  Inductance=1e-3  SetiL0=off  InitialCurrent=0  Capacitance=1e-6  Setx0=off  InitialVoltage=0  Measurements=None
  Rs_ : Gain  Gain=Rs_array
  t0_kW : Gain  Gain=1e-3
  + : PMIOPort  Port=1  Side=Right
  - : PMIOPort  Port=2  Side=Right
  m : Outport
  wires:
  I_PV/1 -> Bus Creator/2, Rs_/1  "I_PV"
  Bus Creator/1 -> m/1
  Rs_/1 -> Add/2
  Diode/1(Vdiode) -> Add/1  "Vdiode"
  Diode/2(Idiode) -> Bus Creator/3  "I_diode"
  Add/1 -> Bus Creator/1  "V_PV"
  t0_kW/1 -> Product1/2
  Product1/1 -> Iph/1
  Iph_/1 -> Product1/1
  Ir/1 -> Bus Creator/4, t0_kW/1
  connections:
  +/RConn1 -- I_PV/RConn1
  Rs/LConn1 -- I_PV/LConn1
  Rp/LConn1 -- Rs/RConn1 -- Iph/RConn1 -- Diode/LConn1
  Rp/RConn1 -- Diode/RConn1 -- Iph/LConn1 -- -/RConn1

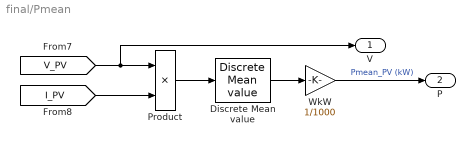
== system final/Pmean ==
  Discrete Mean value : powerlib_extras/Discrete Measurements/Discrete  Mean value  Freq=60  Vinit=0  Ts=Ts_Control
  Product : Product  RndMeth=Zero
  WkW : Gain  Gain=1/1000
  V : Outport
  P : Outport  Port=2
  wires:
  [V_PV] -> Product/1, V/1
  Product/1 -> Discrete Mean value/1
  [I_PV] -> Product/2
  WkW/1 -> P/1  "Pmean_PV (kW)"
  Discrete Mean value/1 -> WkW/1

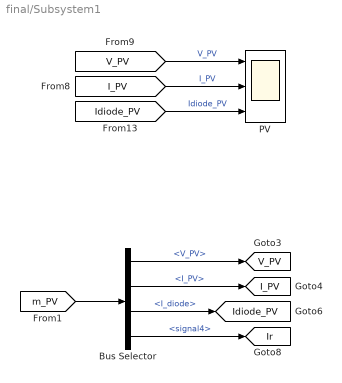
== system final/Subsystem1 ==
  Bus Selector : BusSelector  OutputSignals=V_PV,I_PV,I_diode,signal4
  PV : Scope  NumInputPorts=3
      settings: TimeRange=2  YMin=240~0~0  YMax=280~400~50  SaveName=ScopeData2  Decimation=100
  tag scope: I_PV=global, Idiode_PV=global, Ir=global, V_PV=global
  wires:
  [V_PV] -> PV/1  "V_PV"
  [I_PV] -> PV/2  "I_PV"
  [Idiode_PV] -> PV/3  "Idiode_PV"
  [m_PV] -> Bus Selector/1
  Bus Selector/1 -> [V_PV]  "<V_PV>"
  Bus Selector/2 -> [I_PV]  "<I_PV>"
  Bus Selector/3 -> [Idiode_PV]  "<I_diode>"
  Bus Selector/4 -> [Ir]  "<signal4>"

== system final/Subsystem2 ==
  Discrete Mean value : powerlib_extras/Discrete Measurements/Discrete  Mean value  Freq=60  Vinit=0  Ts=Ts_Control
  Vm : Outport
  wires:
  [Vdc] -> Discrete Mean value/1  "Vdc"
  Discrete Mean value/1 -> Vm/1

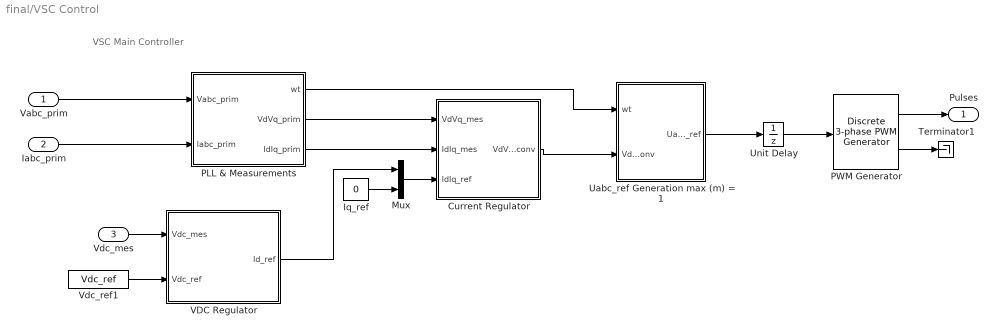
== system final/VSC Control ==
  note: VSC Main Controller
  Vabc_prim : Inport  PortDimensions=3
  Iabc_prim : Inport  Port=2  PortDimensions=3
  Vdc_mes : Inport  Port=3  PortDimensions=1
  Current Regulator : Subsystem
  Iq_ref : Constant  Value=0
  Mux : Mux  Inputs=2
  PLL & Measurements : Subsystem
  PWM Generator : powerlib_extras/Discrete  Control Blocks/Discrete 3-phase PWM Generator  ModulatorType=3-level  ModulatorMode=Un-synchronized  nF=18  Fc=33*60  ModulatingSignals=off  m=0.2  Freq=60  Phase=0  Ts=Ts_Power
  Terminator1 : Terminator
  Uabc_ref Generation max (m) = 1 : Subsystem
  Unit Delay : UnitDelay  SampleTime=Ts_Control
  VDC Regulator : Subsystem
  Vdc_ref1 : Constant  Value=Vdc_ref
  Pulses : Outport
  wires:
  VDC Regulator/1(Id_ref) -> Mux/1
  PLL & Measurements/1(wt) -> Uabc_ref Generation max (m) = 1/1(wt)
  Current Regulator/1(VdVq_conv) -> Uabc_ref Generation max (m) = 1/2(VdVq_conv)
  Iq_ref/1 -> Mux/2
  Mux/1 -> Current Regulator/3(IdIq_ref)
  PLL & Measurements/3(IdIq_prim) -> Current Regulator/2(IdIq_mes)
  PLL & Measurements/2(VdVq_prim) -> Current Regulator/1(VdVq_mes)
  Vdc_mes/1 -> VDC Regulator/1(Vdc_mes)
  Vabc_prim/1 -> PLL & Measurements/1(Vabc_prim)
  Iabc_prim/1 -> PLL & Measurements/2(Iabc_prim)
  Unit Delay/1 -> PWM Generator/1
  PWM Generator/1 -> Pulses/1
  Uabc_ref Generation max (m) = 1/1(Uabc_ref) -> Unit Delay/1
  PWM Generator/2 -> Terminator1/1
  Vdc_ref1/1 -> VDC Regulator/2(Vdc_ref)

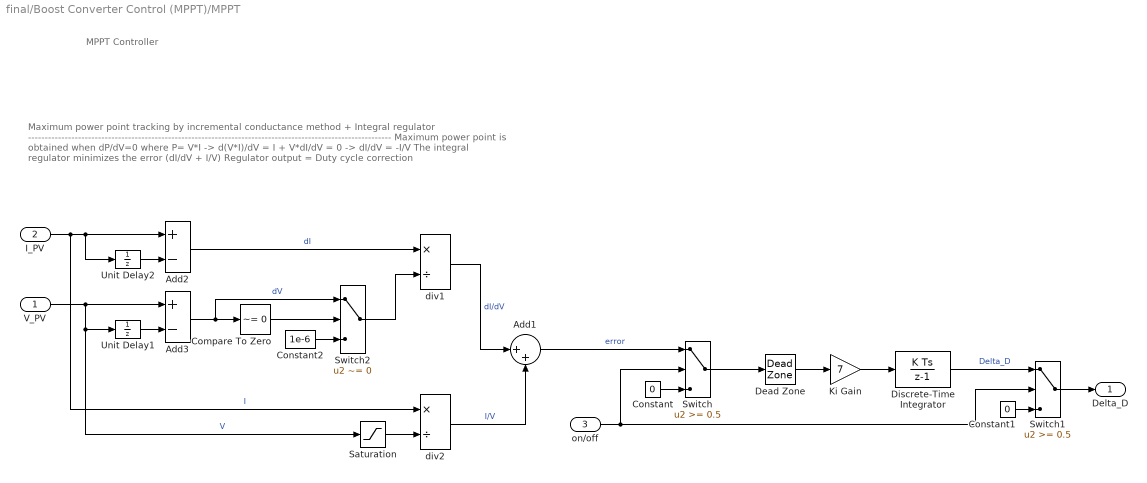
== system final/Boost Converter Control (MPPT)/MPPT ==
  note: Maximum power point tracking by incremental conductance method + Integral regulator
      | -------------------------------------------------------------------------------------------------------------
      | Maximum power point is obtained when dP/dV=0  where P= V*I
      | -> d(V*I)/dV = I + V*dI/dV = 0
      | -> dI/dV = -I/V
      | The integral regulator minimizes the error (dI/dV + I/V)
      | Regulator output = Duty cycle correction
  note: MPPT Controller
  V_PV : Inport
  I_PV : Inport  Port=2
  on/off : Inport  Port=3
  Add1 : Sum  Inputs=|++
  Add2 : Sum  Inputs=+-
  Add3 : Sum  Inputs=+-
  Compare To Zero : simulink/Logic and Bit Operations/Compare To Zero  relop=~=  OutDataTypeStr=uint8
  Constant : Constant  Value=0
  Constant1 : Constant  Value=0
  Constant2 : Constant  Value=1e-6
  Dead Zone : DeadZone  LowerValue=-0.02  UpperValue=+0.02  SaturateOnIntegerOverflow=on
  Discrete-Time Integrator : DiscreteIntegrator  gainval=1  SampleTime=Ts_Control  LimitOutput=on  UpperSaturationLimit=1  LowerSaturationLimit=-1
  Ki Gain : Gain  Gain=7
  Saturation : Saturate  UpperLimit=inf  LowerLimit=eps
  Switch : Switch  Threshold=0.5
  Switch1 : Switch  Threshold=0.5
  Switch2 : Switch  Criteria=u2 ~= 0
  Unit Delay1 : UnitDelay  SampleTime=Ts_Control
  Unit Delay2 : UnitDelay  SampleTime=Ts_Control
  div1 : Product  Inputs=*/  RndMeth=Zero
  div2 : Product  Inputs=*/  RndMeth=Zero
  Delta_D : Outport
  wires:
  V_PV/1 -> Add3/1, Saturation/1, Unit Delay1/1  "V"
  div1/1 -> Add1/1  "dI/dV"
  Constant/1 -> Switch/3
  Switch/1 -> Dead Zone/1
  Unit Delay1/1 -> Add3/2
  Compare To Zero/1 -> Switch2/2
  Switch2/1 -> div1/2
  Constant2/1 -> Switch2/3
  I_PV/1 -> Unit Delay2/1, Add2/1, div2/1  "I"
  Unit Delay2/1 -> Add2/2
  Add3/1 -> Compare To Zero/1, Switch2/1  "dV"
  Add2/1 -> div1/1  "dI"
  Saturation/1 -> div2/2
  div2/1 -> Add1/2  "I/V"
  Add1/1 -> Switch/1  "error"
  Dead Zone/1 -> Ki Gain/1
  Constant1/1 -> Switch1/3
  Discrete-Time Integrator/1 -> Switch1/1  "Delta_D"
  Switch1/1 -> Delta_D/1
  on/off/1 -> Switch/2, Switch1/2
  Ki Gain/1 -> Discrete-Time Integrator/1

== system final/Boost Converter Control (MPPT)/Pulse Generator ==
  D : Inport
  Relational Operator : RelationalOperator  Operator=<=  OutDataTypeStr=boolean
  Repeating Sequence : simulink/Sources/Repeating Sequence  rep_seq_t="[0  1/Freq]"  rep_seq_y=[0 1]
  Pulses : Outport
  wires:
  D/1 -> Relational Operator/2
  Relational Operator/1 -> Pulses/1
  Repeating Sequence/1 -> Relational Operator/1

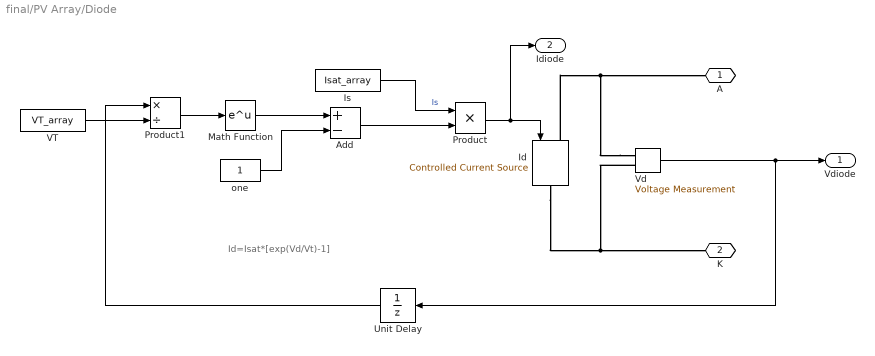
== system final/PV Array/Diode ==
  note: Id=Isat*[exp(Vd/Vt)-1]
  Add : Sum  Inputs=+-
  Id : powerlib/Electrical Sources/Controlled Current Source  Initialize=on  Source_Type=AC  Amplitude=0  Phase=0  Frequency=0  Measurements=None
  Is : Constant  Value=Isat_array
  Math Function : Math  SaturateOnIntegerOverflow=on
  Product : Product  RndMeth=Zero
  Product1 : Product  Inputs=*/  RndMeth=Zero
  Unit Delay : UnitDelay  SampleTime=Ts
  VT : Constant  Value=VT_array
  Vd : powerlib/Measurements/Voltage Measurement  PhasorSimulation=off  OutputType=Complex  PSBequivalent=0
  one : Constant
  A : PMIOPort  Port=1  Side=Left
  K : PMIOPort  Port=2  Side=Right
  Vdiode : Outport
  Idiode : Outport  Port=2
  wires:
  Product/1 -> Idiode/1, Id/1
  Vd/1 -> Vdiode/1, Unit Delay/1
  Is/1 -> Product/1  "Is"
  Product1/1 -> Math Function/1
  one/1 -> Add/2
  Add/1 -> Product/2
  VT/1 -> Product1/2
  Unit Delay/1 -> Product1/1
  Math Function/1 -> Add/1
  connections:
  Id/RConn1 -- K/RConn1 -- Vd/LConn2
  Vd/LConn1 -- A/RConn1 -- Id/LConn1

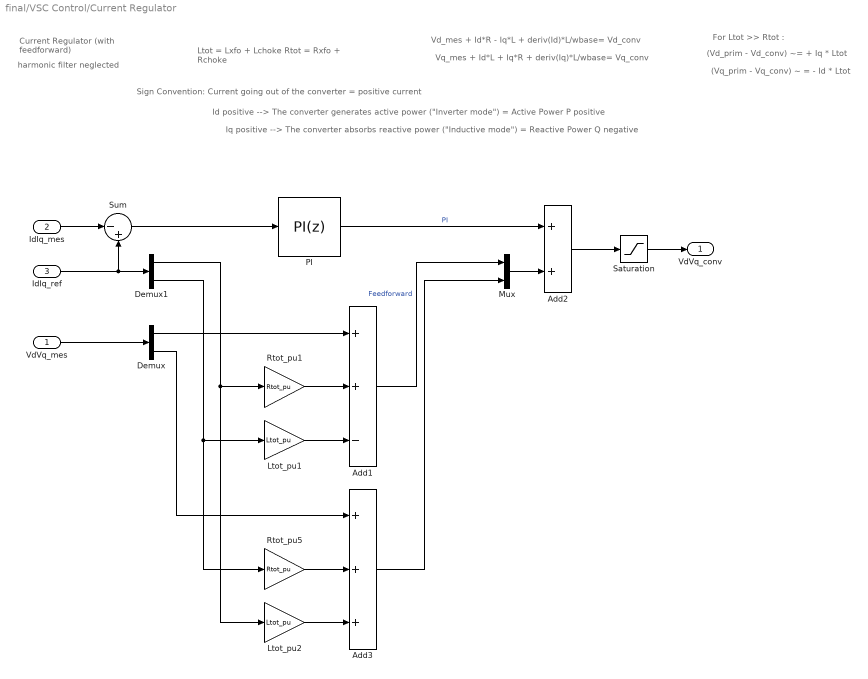
== system final/VSC Control/Current Regulator ==
  note: harmonic filter neglected
  note: Vd_mes + Id*R - Iq*L + deriv(Id)*L/wbase= Vd_conv
  note: Vq_mes + Id*L + Iq*R + deriv(Iq)*L/wbase= Vq_conv
  note: Current Regulator
      | (with feedforward)
  note: Sign Convention: Current going out of the converter = positive current
  note: Iq positive --> The converter absorbs reactive power ("Inductive mode") = Reactive Power Q negative
  note: Id positive --> The converter generates active power ("Inverter mode") = Active Power P positive
  note: Ltot = Lxfo + Lchoke
      | Rtot = Rxfo + Rchoke
  note: (Vd_prim - Vd_conv) ~= + Iq * Ltot
  note: (Vq_prim - Vq_conv) ~ = - Id * Ltot
  note: For Ltot >> Rtot :
  VdVq_mes : Inport  PortDimensions=2
  IdIq_mes : Inport  Port=2  PortDimensions=2
  IdIq_ref : Inport  Port=3  PortDimensions=2
  Add1 : Sum  Inputs=++-
  Add2 : Sum
  Add3 : Sum  Inputs=+++
  Demux : Demux  Outputs=2
  Demux1 : Demux  Outputs=2
  Ltot_pu1 : Gain  Gain=Ltot_pu  SaturateOnIntegerOverflow=on  OutDataTypeStr=Inherit: Same as input  ParamDataTypeStr=Inherit: Same as input
  Ltot_pu2 : Gain  Gain=Ltot_pu  SaturateOnIntegerOverflow=on  OutDataTypeStr=Inherit: Same as input  ParamDataTypeStr=Inherit: Same as input
  Mux : Mux  Inputs=2
  PI : simulink/Continuous/PID Controller  Controller=PI  TimeDomain=Discrete-time  SampleTime=Ts  IntegratorMethod=Forward Euler  FilterMethod=Forward Euler  Form=Parallel  UseFilter=on  ControllerParametersSource=internal  P=Kp_Ireg  I=Ki_Ireg  D=0  N=100  InitialConditionSource=internal  InitialConditionForIntegrator=0  InitialConditionForFilter=0  ExternalReset=none  LimitOutput=on  UpperSaturationLimit=2  LowerSaturationLimit=-2  LinearizeAsGain=off  AntiWindupMode=none  Kb=1  TrackingMode=off  Kt=1  PParamMin=[]  PParamMax=[]  IParamMin=[]  IParamMax=[]  DParamMin=[]  DParamMax=[]  NParamMin=[]  NParamMax=[]  KbParamMin=[]  KbParamMax=[]  KtParamMin=[]  KtParamMax=[]  POutMin=[]  POutMax=[]  IOutMin=[]  IOutMax=[]  DOutMin=[]  DOutMax=[]  NOutMin=[]  NOutMax=[]  KbOutMin=[]  KbOutMax=[]  KtOutMin=[]  KtOutMax=[]  IntegratorOutMin=[]  IntegratorOutMax=[]  FilterOutMin=[]  FilterOutMax=[]  SumOutMin=[]  SumOutMax=[]  SumI1OutMin=[]  SumI1OutMax=[]  SumI2OutMin=[]  SumI2OutMax=[]  SumI3OutMin=[]  SumI3OutMax=[]  SumDOutMin=[]  SumDOutMax=[]  SaturationOutMin=[]  SaturationOutMax=[]  IntegratorContinuousStateAttributes=''  IntegratorStateMustResolveToSignalObject=off  IntegratorRTWStateStorageClass=Auto  FilterContinuousStateAttributes=''  FilterStateMustResolveToSignalObject=off  FilterRTWStateStorageClass=Auto  DifferentiatorICPrevScaledInput=0  DifferentiatorOutMin=[]  DifferentiatorOutMax=[]
  Rtot_pu1 : Gain  Gain=Rtot_pu  SaturateOnIntegerOverflow=on  OutDataTypeStr=Inherit: Same as input  ParamDataTypeStr=Inherit: Same as input
  Rtot_pu5 : Gain  Gain=Rtot_pu  SaturateOnIntegerOverflow=on  OutDataTypeStr=Inherit: Same as input  ParamDataTypeStr=Inherit: Same as input
  Saturation : Saturate  UpperLimit=2  LowerLimit=-2
  Sum : Sum  Inputs=|-+
  VdVq_conv : Outport
  wires:
  Mux/1 -> Add2/2
  PI/1 -> Add2/1  "PI"
  Sum/1 -> PI/1
  IdIq_ref/1 -> Sum/2, Demux1/1
  IdIq_mes/1 -> Sum/1
  Add2/1 -> Saturation/1
  Saturation/1 -> VdVq_conv/1
  VdVq_mes/1 -> Demux/1
  Demux/1 -> Add1/1
  Rtot_pu1/1 -> Add1/2
  Demux1/1 -> Rtot_pu1/1, Ltot_pu2/1
  Ltot_pu1/1 -> Add1/3
  Demux1/2 -> Ltot_pu1/1, Rtot_pu5/1
  Rtot_pu5/1 -> Add3/2
  Ltot_pu2/1 -> Add3/3
  Add1/1 -> Mux/1  "Feedforward"
  Demux/2 -> Add3/1
  Add3/1 -> Mux/2

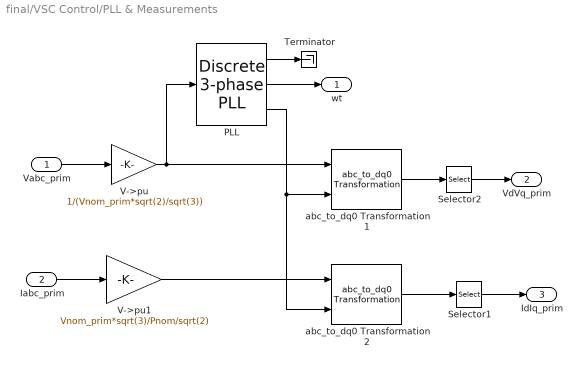
== system final/VSC Control/PLL & Measurements ==
  Vabc_prim : Inport
  Iabc_prim : Inport  Port=2
  PLL : powerlib_extras/Discrete  Control Blocks/Discrete 3-phase PLL  Fmin=45  Par_Init="[-0.57  Fnom]"  ParK=[60 1400]  Ts=Ts  AGC=off
  Selector1 : Selector  InputPortWidth=3  Indices=[1 2]
  Selector2 : Selector  InputPortWidth=3  Indices=[1 2]
  Terminator : Terminator
  V->pu : Gain  Gain=1/(Vnom_prim*sqrt(2)/sqrt(3))  SaturateOnIntegerOverflow=on  OutDataTypeStr=Inherit: Same as input  ParamDataTypeStr=Inherit: Same as input
  V->pu1 : Gain  Gain=Vnom_prim*sqrt(3)/Pnom/sqrt(2)  SaturateOnIntegerOverflow=on  OutDataTypeStr=Inherit: Same as input  ParamDataTypeStr=Inherit: Same as input
  abc_to_dq0 Transformation1 : powerlib_extras/Measurements/abc_to_dq0 Transformation
  abc_to_dq0 Transformation2 : powerlib_extras/Measurements/abc_to_dq0 Transformation
  wt : Outport
  VdVq_prim : Outport  Port=2
  IdIq_prim : Outport  Port=3
  wires:
  V->pu1/1 -> abc_to_dq0 Transformation2/1
  V->pu/1 -> abc_to_dq0 Transformation1/1, PLL/1
  abc_to_dq0 Transformation2/1 -> Selector1/1
  PLL/2 -> wt/1
  Vabc_prim/1 -> V->pu/1
  Iabc_prim/1 -> V->pu1/1
  abc_to_dq0 Transformation1/1 -> Selector2/1
  Selector2/1 -> VdVq_prim/1
  Selector1/1 -> IdIq_prim/1
  PLL/3 -> abc_to_dq0 Transformation2/2, abc_to_dq0 Transformation1/2
  PLL/1 -> Terminator/1

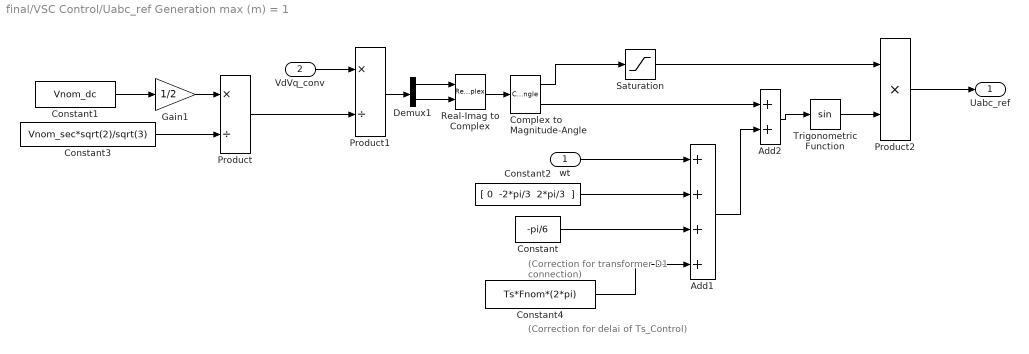
== system final/VSC Control/Uabc_ref Generation max (m) = 1 ==
  note: (Correction for transformer
      |  D1 connection)
  note: (Correction for delai of Ts_Control)
  wt : Inport
  VdVq_conv : Inport  Port=2
  Add1 : Sum  Inputs=++++
  Add2 : Sum
  Complex to Magnitude-Angle : ComplexToMagnitudeAngle
  Constant : Constant  Value=-pi/6
  Constant1 : Constant  Value=Vnom_dc
  Constant2 : Constant  Value="[ 0  -2*pi/3  2*pi/3  ]"
  Constant3 : Constant  Value=Vnom_sec*sqrt(2)/sqrt(3)
  Constant4 : Constant  Value=Ts*Fnom*(2*pi)
  Demux1 : Demux  Outputs=2
  Gain1 : Gain  Gain=1/2
  Product : Product  Inputs=*/  RndMeth=Zero
  Product1 : Product  Inputs=*/  RndMeth=Zero
  Product2 : Product  Inputs=**  RndMeth=Zero
  Real-Imag to Complex : RealImagToComplex
  Saturation : Saturate  UpperLimit=1  LowerLimit=0
  Trigonometric Function : Trigonometry
  Uabc_ref : Outport
  wires:
  Complex to Magnitude-Angle/1 -> Saturation/1
  Constant1/1 -> Gain1/1
  VdVq_conv/1 -> Product1/1
  Product1/1 -> Demux1/1
  Gain1/1 -> Product/1
  Real-Imag to Complex/1 -> Complex to Magnitude-Angle/1
  Demux1/1 -> Real-Imag to Complex/1
  Demux1/2 -> Real-Imag to Complex/2
  Constant2/1 -> Add1/2
  Constant/1 -> Add1/3
  Constant3/1 -> Product/2
  Product/1 -> Product1/2
  Complex to Magnitude-Angle/2 -> Add2/1
  Add1/1 -> Add2/2
  Add2/1 -> Trigonometric Function/1
  Saturation/1 -> Product2/1
  Trigonometric Function/1 -> Product2/2
  Product2/1 -> Uabc_ref/1
  wt/1 -> Add1/1
  Constant4/1 -> Add1/4
